simulink model "sampleModel1649_2_sub_sub"  (R2023a)
settings: Solver=VariableStepAuto  StartTime=0.0  StopTime=10.0  RelTol=1e-3
libraries: simulink x6, hdlsllib x5
settings Model: Creator=user1  LastModifiedBy=user1
settings OptimizationCC: BlockReduction=off  ConditionallyExecuteInputs=off

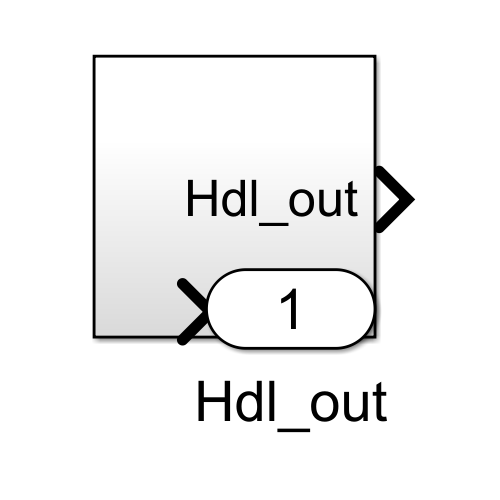
[thumbnail: Simulink's stored preview of the top-level diagram]
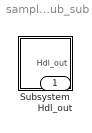
== system sampleModel1649_2_sub_sub ==
  Subsystem : Subsystem
  Hdl_out : Outport  OutDataTypeStr=uint8

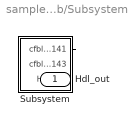
== system sampleModel1649_2_sub_sub/Subsystem ==
  Subsystem : Subsystem
  Hdl_out : Outport  OutDataTypeStr=uint8
  wires:
  Subsystem/1(cfblk141) -> Hdl_out/1

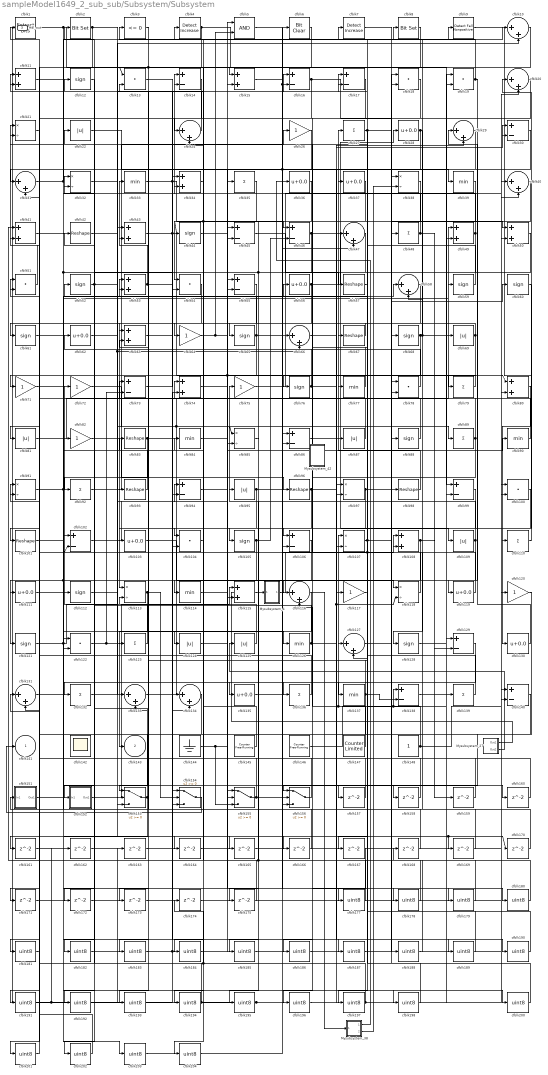
== system sampleModel1649_2_sub_sub/Subsystem/Subsystem ==
  Mysubsystem_27 : Subsystem  TreatAsAtomicUnit=on  RTWFcnName=Mysubsystem_27
      settings: RTWFcnNameOpts=User specified  RTWFileNameOpts=Use function name
  Mysubsystem_38 : Subsystem  TreatAsAtomicUnit=on  RTWFcnName=Mysubsystem_38
      settings: RTWFcnNameOpts=User specified  RTWFileNameOpts=Use function name
  Mysubsystem_4 : Subsystem  TreatAsAtomicUnit=on  RTWFcnName=Mysubsystem_4
      settings: RTWFcnNameOpts=User specified  RTWFileNameOpts=Use function name
  Mysubsystem_42 : Subsystem  TreatAsAtomicUnit=on  RTWFcnName=Mysubsystem_42
      settings: RTWFcnNameOpts=User specified  RTWFileNameOpts=Use function name
  cfblk1 : simulink/Logic and Bit Operations/Extract Bits  bitsToExtract=Upper half  numBits=8  bitIdxRange=[0 7]  outScalingMode=Preserve fixed-point scaling
      settings: LibrarySourceBlock=|
      | hdlsllib/Logic and Bit
      | Operations/Extract Bits
  cfblk{10,20,24,29,31,40,47,58,66,116,127,131,133..134} (14 alike) : Sum  Inputs=|++  OutDataTypeStr=uint8
  cfblk{13,18..19,51,54,78,100,104,122} (9 alike) : DotProduct  OutDataTypeStr=uint8
  cfblk{42,57,67,83,93,96,98,101} (8 alike) : Reshape
  cfblk{14,16..17,30,45..46,55,73,86,94,99,102,106,129,138,140} (16 alike) : Sum  Inputs=+-  OutDataTypeStr=uint8
  cfblk{28,36..37,56,62,103,111,119,130,135} (10 alike) : Bias  Bias=0.0  SaturateOnIntegerOverflow=off
  cfblk{12,44,52,59..61,65,68,76,88,105,112,121,128} (14 alike) : Signum
  cfblk{21,32,38,85,91,97,107,113,118} (9 alike) : Product  Inputs=*/  OutDataTypeStr=uint8  RndMeth=Zero  SaturateOnIntegerOverflow=on
  cfblk{11,15,34,41,43,49..50,53,63,74,80,108,115} (13 alike) : Sum  OutDataTypeStr=uint8
  cfblk{22,69,81,87,95,109,124..125} (8 alike) : Abs  OutDataTypeStr=uint8  SaturateOnIntegerOverflow=off
  cfblk{27,35,48,79,89,92,110,123,132,136,139} (11 alike) : Sum  Inputs=+  OutDataTypeStr=uint8
  cfblk{33,39,77,84,90,114,126,137} (8 alike) : MinMax  OutDataTypeStr=uint8
  cfblk{26,64,71..72,75,82,117,120} (8 alike) : Gain  OutDataTypeStr=uint8
  cfblk142 : Scope
      settings: Floating=on
  cfblk144 : Ground
  cfblk145 : hdlsllib/Sources/Counter Free-Running  NumBits=16  tsamp=-1
  cfblk146 : hdlsllib/Sources/Counter Free-Running  NumBits=16  tsamp=-1
  cfblk147 : hdlsllib/Sources/Counter Limited  uplimit=7  tsamp=-1
  cfblk148 : Constant  OutDataTypeStr=uint8  SampleTime=-1
  cfblk151 : Subsystem
      settings: LibrarySourceBlock=|
      | hdlsllib/Ports &
      | Subsystems/Subsystem
  cfblk152 : Subsystem
      settings: LibrarySourceBlock=|
      | hdlsllib/Ports &
      | Subsystems/Subsystem
  cfblk{153..156} (4 alike) : Switch  OutDataTypeStr=uint8  SaturateOnIntegerOverflow=off  InputSameDT=off
  cfblk{157..175} (19 alike) : Delay  SampleTime=1
  cfblk{177..198,200..204} (27 alike) : DataTypeConversion  OutDataTypeStr=uint8  SaturateOnIntegerOverflow=off  RndMeth=Floor
  cfblk2 : simulink/Logic and Bit Operations/Bit Set  iBit=0
      settings: LibrarySourceBlock=|
      | hdlsllib/Logic and Bit
      | Operations/Bit Set
  cfblk3 : hdlsllib/Logic and Bit Operations/Compare To Zero  relop=<=  OutDataTypeStr=uint8
  cfblk4 : simulink/Logic and Bit Operations/Detect Increase  vinit=0.0  OutDataTypeStr=uint8
      settings: LibrarySourceBlock=|
      | hdlsllib/Logic and Bit
      | Operations/Detect
      | Increase
  cfblk5 : Logic  AllPortsSameDT=off  OutDataTypeStr=boolean
  cfblk6 : simulink/Logic and Bit Operations/Bit Clear  iBit=0
      settings: LibrarySourceBlock=|
      | hdlsllib/Logic and Bit
      | Operations/Bit Clear
  cfblk7 : simulink/Logic and Bit Operations/Detect Increase  vinit=0.0  OutDataTypeStr=uint8
      settings: LibrarySourceBlock=|
      | hdlsllib/Logic and Bit
      | Operations/Detect
      | Increase
  cfblk8 : simulink/Logic and Bit Operations/Bit Set  iBit=0
      settings: LibrarySourceBlock=|
      | hdlsllib/Logic and Bit
      | Operations/Bit Set
  cfblk9 : hdlsllib/Logic and Bit Operations/Detect Fall Nonpositive  vinit=0  OutDataTypeStr=uint8
  cfblk141 : Outport  OutDataTypeStr=uint8  VectorParamsAs1DForOutWhenUnconnected=off
  cfblk143 : Outport  Port=2  OutDataTypeStr=uint8  VectorParamsAs1DForOutWhenUnconnected=off
  Hdl_out : Outport  Port=3  OutDataTypeStr=uint8
  wires:
  Mysubsystem_38/2(Out2) -> cfblk38/2
  Mysubsystem_38/1(Out1) -> cfblk36/1
  Mysubsystem_4/1(Out1) -> Mysubsystem_38/1(In1)
  Mysubsystem_27/2(Out2) -> cfblk125/1
  Mysubsystem_27/1(Out1) -> Mysubsystem_4/1(In1)
  cfblk204/1 -> cfblk86/2
  cfblk6/1 -> cfblk204/1
  cfblk203/1 -> cfblk6/1
  cfblk202/1 -> cfblk131/2
  cfblk12/1 -> cfblk202/1
  cfblk201/1 -> cfblk131/1
  cfblk200/1 -> cfblk67/1
  cfblk131/1 -> cfblk200/1
  cfblk198/1 -> cfblk38/1
  cfblk61/1 -> cfblk198/1
  cfblk197/1 -> cfblk174/1, cfblk112/1, cfblk129/1
  cfblk196/1 -> cfblk140/2
  cfblk167/1 -> cfblk196/1
  cfblk195/1 -> cfblk140/1, Hdl_out/1
  cfblk194/1 -> cfblk51/2, cfblk97/1
  cfblk193/1 -> cfblk134/2
  cfblk192/1 -> cfblk134/1
  cfblk14/1 -> cfblk192/1
  cfblk191/1 -> cfblk163/1, cfblk162/1
  cfblk190/1 -> cfblk127/2
  cfblk189/1 -> cfblk127/1
  cfblk66/1 -> cfblk189/1
  cfblk188/1 -> cfblk168/1
  cfblk127/1 -> cfblk188/1
  cfblk187/1 -> cfblk40/2
  cfblk186/1 -> cfblk40/1
  cfblk185/1 -> cfblk100/1
  cfblk40/1 -> cfblk185/1
  cfblk184/1 -> cfblk55/2
  cfblk183/1 -> cfblk55/1
  cfblk182/1 -> cfblk154/1, cfblk68/1
  cfblk181/1 -> cfblk41/2
  cfblk180/1 -> cfblk41/1
  cfblk7/1 -> cfblk180/1
  cfblk179/1 -> cfblk52/1
  cfblk41/1 -> cfblk179/1
  cfblk178/1 -> cfblk84/1
  cfblk177/1 -> cfblk31/2, cfblk95/1
  cfblk175/1 -> cfblk91/2
  cfblk174/1 -> cfblk50/2
  cfblk173/1 -> cfblk80/2
  cfblk172/1 -> cfblk74/2
  cfblk129/1 -> cfblk172/1
  cfblk171/1 -> cfblk97/2
  cfblk170/1 -> cfblk108/2
  cfblk169/1 -> cfblk155/1
  cfblk168/1 -> cfblk122/1
  cfblk166/1 -> cfblk43/2
  cfblk165/1 -> cfblk18/1
  cfblk63/1 -> cfblk165/1
  cfblk164/1 -> cfblk106/2
  cfblk101/1 -> cfblk164/1
  cfblk163/1 -> cfblk99/2
  cfblk162/1 -> cfblk47/1
  cfblk161/1 -> cfblk100/2
  cfblk160/1 -> cfblk133/2
  cfblk94/1 -> cfblk160/1
  cfblk159/1 -> cfblk19/1
  cfblk158/1 -> cfblk86/1
  cfblk114/1 -> cfblk158/1
  cfblk157/1 -> cfblk1/1
  cfblk36/1 -> cfblk44/1, cfblk184/1
  cfblk30/1 -> cfblk45/2
  cfblk62/1 -> cfblk10/2
  cfblk96/1 -> cfblk29/2, cfblk175/1
  cfblk13/1 -> cfblk94/2
  cfblk118/1 -> cfblk56/1
  cfblk39/1 -> cfblk58/2
  cfblk10/1 -> cfblk13/1, cfblk183/1
  cfblk69/1 -> cfblk64/1, cfblk123/1
  cfblk32/1 -> cfblk169/1, cfblk170/1, cfblk66/2
  cfblk121/1 -> cfblk43/1, cfblk187/1
  cfblk137/1 -> cfblk153/1, cfblk138/2, cfblk13/2
  cfblk58/1 -> cfblk63/1
  cfblk107/1 -> cfblk18/2, cfblk137/1
  cfblk78/1 -> cfblk62/1
  cfblk87/1 -> cfblk51/1
  cfblk34/1 -> cfblk104/1
  cfblk17/1 -> cfblk24/1
  cfblk37/1 -> cfblk46/1
  cfblk24/1 -> cfblk11/2
  cfblk151/1(Out1) -> cfblk58/1
  cfblk124/1 -> cfblk90/1
  cfblk106/1 -> cfblk122/2, cfblk161/1
  cfblk33/1 -> cfblk156/3, cfblk190/1
  cfblk59/1 -> cfblk22/1
  cfblk2/1 -> cfblk71/1, cfblk166/1
  cfblk119/1 -> cfblk91/1
  cfblk73/1 -> cfblk34/1
  cfblk57/1 -> cfblk37/1
  cfblk29/1 -> cfblk156/2, cfblk173/1
  cfblk139/1 -> cfblk53/1, cfblk102/2
  cfblk16/1 -> cfblk78/1, cfblk154/3
  cfblk72/1 -> cfblk98/1
  cfblk83/1 -> cfblk66/1, cfblk85/1, cfblk92/1
  cfblk15/1 -> cfblk47/2
  cfblk134/1 -> cfblk191/1
  cfblk20/1 -> cfblk116/1
  cfblk100/1 -> cfblk103/1
  cfblk64/1 -> cfblk5/1, cfblk5/2
  cfblk128/1 -> cfblk69/1
  cfblk122/1 -> cfblk124/1, cfblk73/2
  cfblk85/1 -> cfblk135/1
  cfblk88/1 -> cfblk14/2
  cfblk50/1 -> cfblk193/1, cfblk195/1
  cfblk65/1 -> cfblk101/1, cfblk2/1, cfblk78/2
  cfblk136/1 -> cfblk11/1
  cfblk154/1 -> cfblk141/1
  cfblk145/1 -> cfblk83/1
  cfblk67/1 -> cfblk65/1
  cfblk98/1 -> cfblk87/1
  cfblk52/1 -> cfblk132/1, cfblk85/2
  cfblk144/1 -> cfblk45/1, cfblk155/3
  cfblk79/1 -> cfblk76/1
  cfblk126/1 -> cfblk117/1, cfblk118/2, cfblk102/1
  cfblk76/1 -> cfblk42/1, cfblk30/1
  cfblk132/1 -> cfblk94/1
  cfblk74/1 -> cfblk15/2, cfblk80/1
  cfblk84/1 -> cfblk177/1
  cfblk130/1 -> cfblk29/1
  cfblk117/1 -> cfblk7/1
  cfblk31/1 -> cfblk10/1, cfblk34/2
  cfblk55/1 -> cfblk182/1
  cfblk42/1 -> cfblk133/1
  cfblk115/1 -> cfblk88/1
  cfblk1/1 -> cfblk99/1, cfblk126/1
  cfblk11/1 -> cfblk54/2, cfblk155/2
  cfblk75/1 -> cfblk20/2
  cfblk140/1 -> cfblk194/1
  cfblk49/1 -> cfblk114/1, cfblk24/2
  cfblk110/1 -> cfblk20/1
  cfblk104/1 -> cfblk4/1
  cfblk35/1 -> cfblk54/1
  cfblk8/1 -> cfblk15/1
  cfblk135/1 -> cfblk9/1
  cfblk155/1 -> cfblk108/1, cfblk32/2
  cfblk45/1 -> cfblk57/1
  cfblk102/1 -> cfblk35/1
  cfblk125/1 -> cfblk113/2
  cfblk95/1 -> cfblk77/1, cfblk104/2
  cfblk21/1 -> cfblk61/1
  cfblk153/1 -> cfblk32/1, cfblk171/1
  cfblk60/1 -> cfblk110/1
  cfblk156/1 -> cfblk73/1
  cfblk120/1 -> cfblk156/1
  cfblk68/1 -> cfblk8/1, cfblk30/2, cfblk167/1
  cfblk146/1 -> cfblk49/2, cfblk138/1
  cfblk27/1 -> cfblk50/1, cfblk157/1
  cfblk89/1 -> cfblk136/1, cfblk63/2
  cfblk82/1 -> cfblk96/1
  cfblk71/1 -> cfblk59/1
  cfblk4/1 -> cfblk48/1, cfblk201/1
  cfblk113/1 -> cfblk143/1, cfblk154/2
  cfblk26/1 -> cfblk31/1
  cfblk56/1 -> cfblk28/1, cfblk111/1
  cfblk133/1 -> cfblk19/2
  cfblk51/1 -> cfblk21/2
  cfblk18/1 -> cfblk81/1
  cfblk138/1 -> cfblk139/1
  cfblk19/1 -> cfblk119/1, cfblk3/1
  cfblk28/1 -> cfblk107/2, cfblk128/1
  cfblk123/1 -> cfblk12/1
  cfblk43/1 -> cfblk79/1, cfblk17/2
  cfblk46/1 -> cfblk109/1, cfblk153/3
  cfblk48/1 -> cfblk14/1, cfblk129/2
  cfblk38/1 -> cfblk197/1
  cfblk105/1 -> cfblk121/1, cfblk46/2
  cfblk99/1 -> cfblk105/1
  cfblk5/1 -> cfblk16/2, cfblk178/1
  cfblk3/1 -> cfblk93/1
  cfblk112/1 -> cfblk16/1
  cfblk53/1 -> cfblk33/1, cfblk89/1
  cfblk116/1 -> cfblk151/1(In1)
  cfblk92/1 -> cfblk26/1
  cfblk44/1 -> cfblk115/2
  cfblk148/1 -> cfblk120/1, cfblk17/1
  cfblk108/1 -> cfblk159/1, cfblk181/1
  cfblk111/1 -> cfblk82/1
  cfblk103/1 -> cfblk118/1
  cfblk54/1 -> cfblk113/1
  cfblk80/1 -> cfblk130/1
  cfblk22/1 -> cfblk39/1
  cfblk81/1 -> cfblk49/1
  cfblk147/1 -> cfblk107/1, cfblk116/2
  cfblk97/1 -> cfblk60/1, cfblk186/1
  cfblk152/1(Out1) -> cfblk115/1
  cfblk47/1 -> cfblk152/1(In1)
  cfblk109/1 -> cfblk75/1, cfblk153/2
  cfblk91/1 -> cfblk53/2, cfblk203/1
  cfblk93/1 -> cfblk72/1
  cfblk86/1 -> cfblk27/1
  cfblk9/1 -> cfblk106/1
  cfblk77/1 -> cfblk21/1
  cfblk90/1 -> cfblk74/1

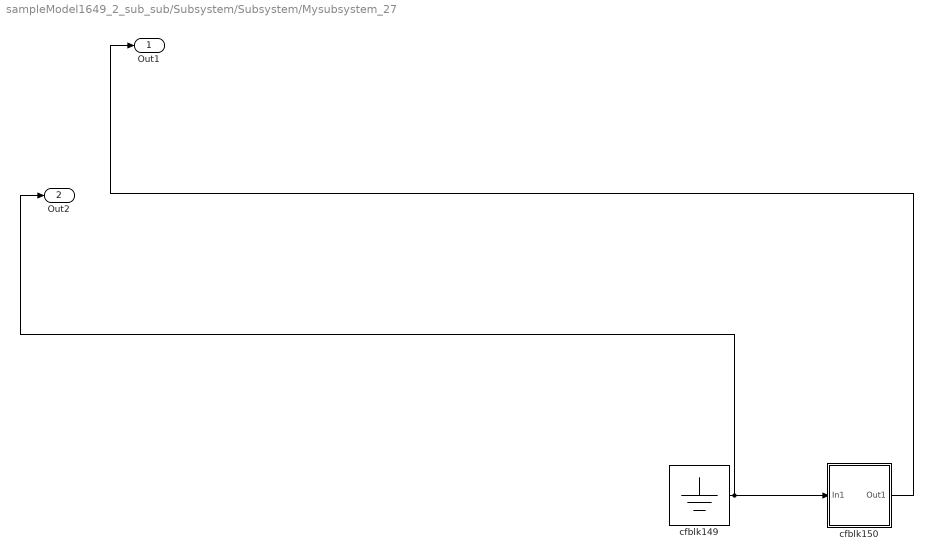
== system sampleModel1649_2_sub_sub/Subsystem/Subsystem/Mysubsystem_27 ==
  cfblk149 : Ground
  cfblk150 : Subsystem
      settings: LibrarySourceBlock=|
      | hdlsllib/Ports &
      | Subsystems/Subsystem
  Out1 : Outport
  Out2 : Outport  Port=2
  wires:
  cfblk149/1 -> Out2/1, cfblk150/1(In1)
  cfblk150/1(Out1) -> Out1/1

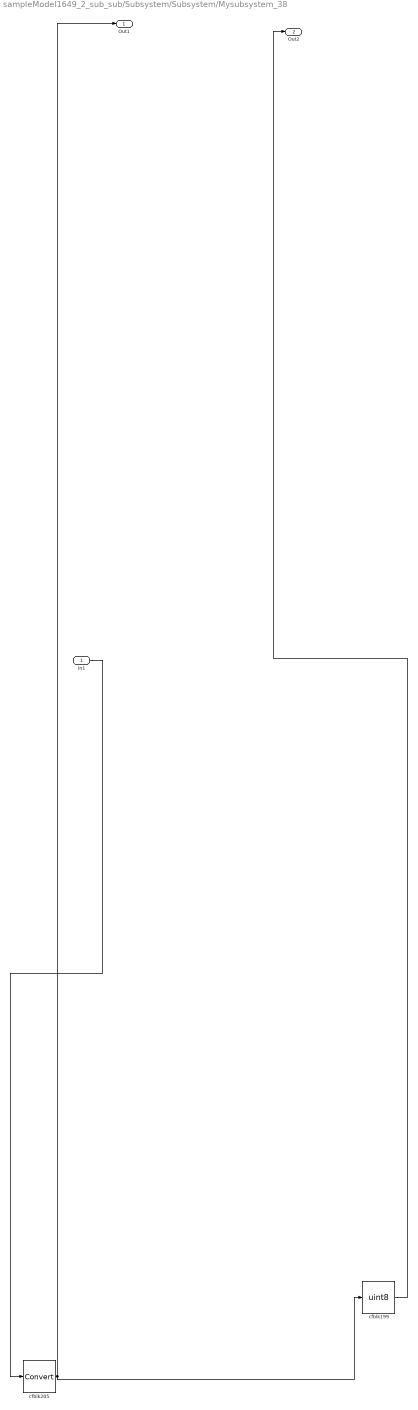
== system sampleModel1649_2_sub_sub/Subsystem/Subsystem/Mysubsystem_38 ==
  In1 : Inport
  cfblk199 : DataTypeConversion  OutDataTypeStr=uint8  SaturateOnIntegerOverflow=off  RndMeth=Floor
  cfblk205 : DataTypeConversion  SaturateOnIntegerOverflow=off  RndMeth=Floor
  Out1 : Outport
  Out2 : Outport  Port=2
  wires:
  cfblk205/1 -> Out1/1, cfblk199/1
  cfblk199/1 -> Out2/1
  In1/1 -> cfblk205/1

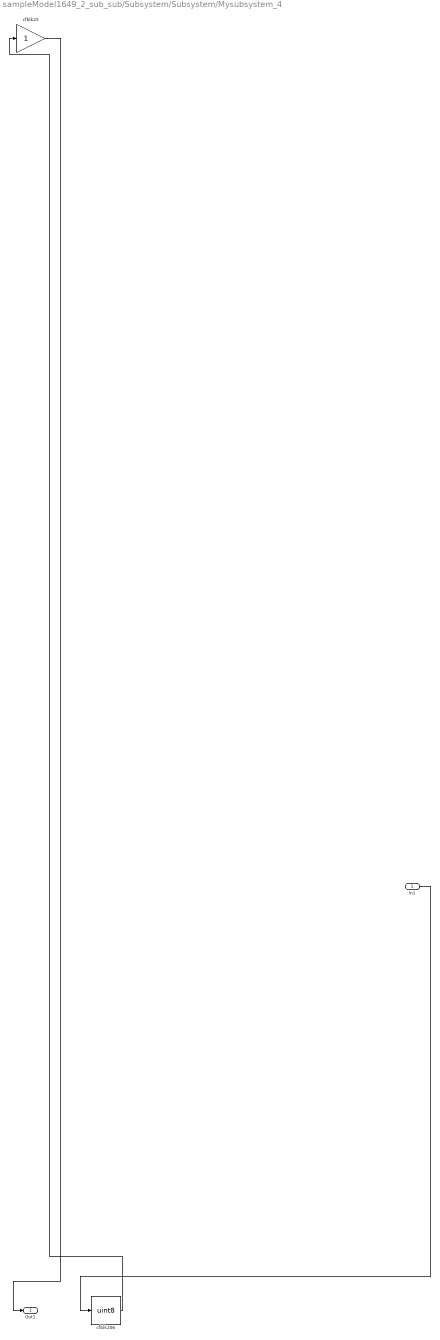
== system sampleModel1649_2_sub_sub/Subsystem/Subsystem/Mysubsystem_4 ==
  In1 : Inport
  cfblk206 : DataTypeConversion  OutDataTypeStr=uint8  SaturateOnIntegerOverflow=off  RndMeth=Floor
  cfblk25 : Gain
  Out1 : Outport
  wires:
  cfblk25/1 -> Out1/1
  cfblk206/1 -> cfblk25/1
  In1/1 -> cfblk206/1

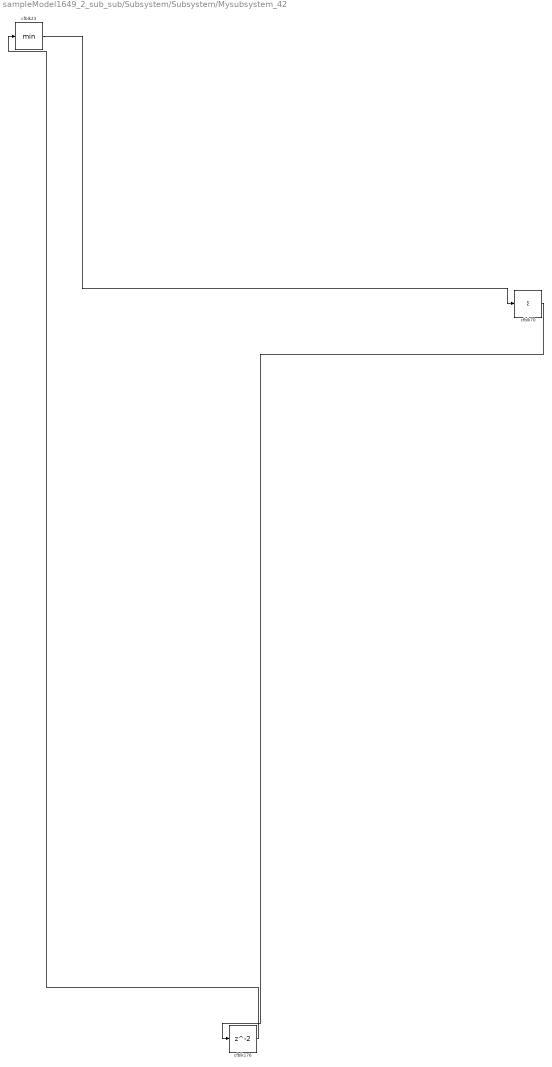
== system sampleModel1649_2_sub_sub/Subsystem/Subsystem/Mysubsystem_42 ==
  cfblk176 : Delay  SampleTime=1
  cfblk23 : MinMax
  cfblk70 : Sum  Inputs=+
  wires:
  cfblk70/1 -> cfblk176/1
  cfblk23/1 -> cfblk70/1
  cfblk176/1 -> cfblk23/1

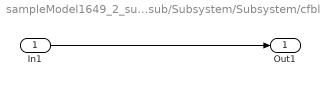
== system sampleModel1649_2_sub_sub/Subsystem/Subsystem/cfblk151 ==
  In1 : Inport
  Out1 : Outport
  wires:
  In1/1 -> Out1/1

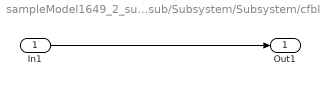
== system sampleModel1649_2_sub_sub/Subsystem/Subsystem/cfblk152 ==
  In1 : Inport
  Out1 : Outport
  wires:
  In1/1 -> Out1/1

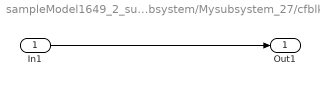
== system sampleModel1649_2_sub_sub/Subsystem/Subsystem/Mysubsystem_27/cfblk150 ==
  In1 : Inport
  Out1 : Outport
  wires:
  In1/1 -> Out1/1
